simulink model "DC_DC_BuckConverter"  (R2016b)
settings: Solver=ode23t  StartTime=0.0  StopTime=0.004  MaxStep=1.e-07  MinStep=1.e-10  RelTol=1e-3  EnableMultiTasking=on
libraries: powerlib x9, simulink x1
settings Model: Creator=sc  LastModifiedBy=Osman Kukrer
settings SolverCC: InitialStep=1.e-07
settings DataIOCC: LimitDataPoints=on  SaveFormat=Array  SignalLoggingSaveFormat=ModelDataLogs
settings OptimizationCC: ExpressionDepthLimit=2147483647  InitFltsAndDblsToZero=on  LifeSpan=inf
settings DebuggingCC: UnderspecifiedInitializationDetection=Classic  MergeDetectMultiDrivingBlocksExec=none  SolverPrmCheckMsg=warning  FcnCallInpInsideContextMsg=warning  StateNameClashWarn=warning  SFUnexpectedBacktrackingDiag=warning  SFNoUnconditionalDefaultTransitionDiag=warning  SFExecutionAtInitializationDiag=none
settings HardwareCC: ProdBitPerPointer=32  ProdBitPerSizeT=32  ProdBitPerPtrDiffT=32  ProdLargestAtomicFloat=None  ProdIntDivRoundTo=Undefined  ProdEndianess=Unspecified  ProdWordSize=32  ProdHWDeviceType=32-bit Generic
settings ModelReferenceCC: PropagateSignalLabelsOutOfModel=off
settings GRTTargetCC: TargetLangStandard=C89/C90 (ANSI)  GeneratePreprocessorConditionals=Disable all  CombineOutputUpdateFcns=off  GRTInterface=on
settings ConfigComp: CovMetricSettings=dw  CovHtmlReporting=on  CovSaveCumulativeToWorkspaceVar=on  CovSaveSingleToWorkspaceVar=on  CovExternalEMLEnable=off

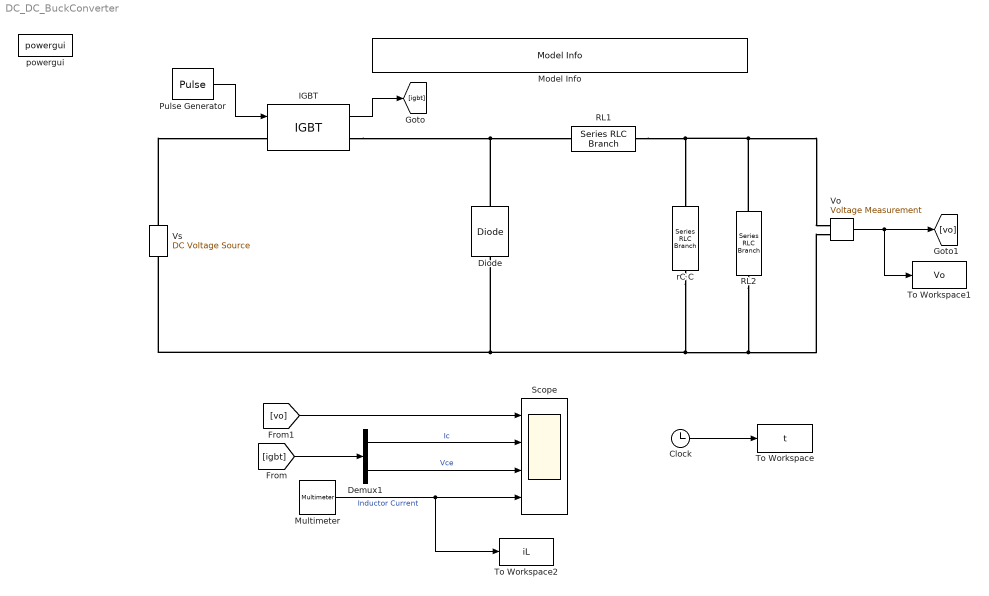
== system DC_DC_BuckConverter ==
  " RL1" : powerlib/Elements/Series RLC Branch  LConnTagsString=__new0  RConnTagsString=__new0  BranchType=L  Resistance=1.0  Inductance=250.e-6  SetiL0=off  InitialCurrent=0  Capacitance=1.0  Setx0=off  InitialVoltage=0  Measurements=Branch current
  " RL2" : powerlib/Elements/Series RLC Branch  LConnTagsString=__new0  RConnTagsString=__new0  BranchType=R  Resistance=10  Inductance=1e-3  SetiL0=off  InitialCurrent=0  Capacitance=1.e-04  Setx0=off  InitialVoltage=0  Measurements=Branch current
  " rC C" : powerlib/Elements/Series RLC Branch  LConnTagsString=__new0  RConnTagsString=__new0  BranchType=RC  Resistance=0.01  Inductance=1e-3  SetiL0=off  InitialCurrent=0  Capacitance=20.e-06  Setx0=off  InitialVoltage=0  Measurements=Branch current
  Clock : Clock
  Demux1 : Demux  Outputs=2
  Diode : powerlib/Power Electronics/Diode  Ron=0.01  Lon=0  Vf=0.8  IC=0  UseSnubber=off  Rs=1000  Cs=inf  Measurements=off
  IGBT : powerlib/Power Electronics/IGBT  Ron=0.001  Lon=0  Vf=0  Tf=1e-7  Tt=1e-7  IC=0  Rs=100  Cs=2.e-08  Measurements=on
  Model Info : simulink/Model-Wide Utilities/Model Info  BlockCM=None  Frame=on  DisplayStringWithTags=DC-DC Buck Converter (DC-DC Step-down converter)  HorizontalTextAlignment=Center  LeftAlignmentValue=0.5  SourceBlockDiagram=DC_DC_BuckConverter  TagMaxNumber=20
  Multimeter : powerlib/Measurements/Multimeter  PhasorSimulation=off  OutputType=Complex  sel=1  L=3  Gain=1  yselected="{'Ib:  RL1'};"  PSBOutputType=1  PSBequivalent=0  AxesSetting=[0,0.1,-100,100]  Display=0  SavedBlockNames=-11
  Pulse Generator : DiscretePulseGenerator  PulseType=Time based  Period=5.e-05  PulseWidth=60
  Scope : Scope  NumInputPorts=4
  To Workspace : ToWorkspace  VariableName=t  SampleTime=-1
  To Workspace1 : ToWorkspace  VariableName=Vo  SampleTime=-1
  To Workspace2 : ToWorkspace  VariableName=iL  SampleTime=-1
  Vo : powerlib/Measurements/Voltage Measurement  PhasorSimulation=off  OutputType=Complex  PSBequivalent=0
  Vs : powerlib/Electrical Sources/DC Voltage Source  Amplitude=100  Measurements=None
  powergui : powerlib/powergui  SimulationMode=Continuous  SolverType=Tustin  SampleTime=50e-6  frequency=60  SPID=off  DisableSnubberDevices=off  DisableRonSwitches=off  DisableVfSwitches=off  SwTol=0  DisplayEquations=off  Interpol=off  ExternalGateDelay=off  methode=off  Ts=0  FunctionMessages=off  echomessages=off  HookPort=off  EnableUseOfTLC=off  x0status=blocks  frequencyindice=0  Pbase=100e6  ErrMax=1e-4  Iterations=50  UnitsV=kV  UnitsW=MW  buscounter=0  RestoreLinks=warning  ResistiveCurrentMeasurement=off  Frange=[0:2:500]  Ylog=off  Xlog=on  ShowGrid=off  save=off  variable=ZData  structure=0  ZoomFFT=on  StartTime=0.0  cycles=1  DisplayStyle=1  fundamental=60  FreqAxis=off  MaxFrequency=1000  frequencyindicesteady=1  RmsSteady=1  display=off
  wires:
  [igbt] -> Demux1/1
  Vo/1 -> [vo], To Workspace1/1
  [vo] -> Scope/1
  Demux1/1 -> Scope/2  "Ic"
  Demux1/2 -> Scope/3  "Vce"
  Multimeter/1 -> Scope/4, To Workspace2/1  "Inductor Current"
  Clock/1 -> To Workspace/1
  IGBT/1 -> [igbt]
  Pulse Generator/1 -> IGBT/1
  connections:
  Vo/LConn2 -- " RL2"/RConn1 -- " rC C"/RConn1 -- Vs/LConn1 -- Diode/LConn1
  " RL2"/LConn1 -- Vo/LConn1 -- " rC C"/LConn1 -- " RL1"/RConn1
  Vs/RConn1 -- IGBT/LConn1
  IGBT/RConn1 -- " RL1"/LConn1 -- Diode/RConn1
